simulink model "chap3_7sim"  (Simulink 7.7)
settings: Solver=ode45  SolverMode=SingleTasking  StartTime=0.0  StopTime=10  FixedStep=0.001  RelTol=1e-3
settings Model: Creator=ljk  LastModifiedBy=ljk  ExtModeTrigMode=oneshot  ExtModeArmWhenConnect=off
settings DataIOCC: LimitDataPoints=off
settings OptimizationCC: BlockReduction=off  BooleanDataType=off
settings DebuggingCC: SaveWithParameterizedLinksMsg=none  SignalResolutionControl=TryResolveAllWithWarning  SolverPrmCheckMsg=none  MultiTaskDSMMsg=warning  MultiTaskCondExecSysMsg=none  StrictBusMsg=None
settings HardwareCC: TargetUnknown=on
settings RTWCC: IncludeERTFirstTime=on

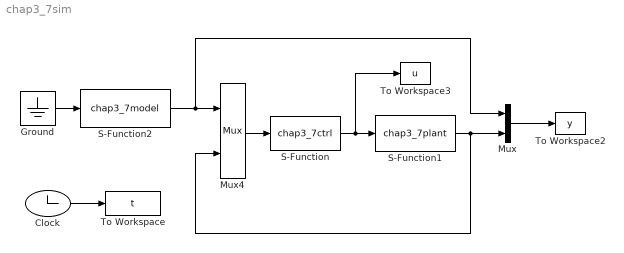
== system chap3_7sim ==
  Clock : Clock
  Ground : Ground
  Mux : Mux  Inputs=2
  Mux4 : Mux  Inputs=2
  S-Function : S-Function  FunctionName=chap3_7ctrl  EnableBusSupport=off
  S-Function1 : S-Function  FunctionName=chap3_7plant  EnableBusSupport=off
  S-Function2 : S-Function  FunctionName=chap3_7model  EnableBusSupport=off
  To Workspace : ToWorkspace  VariableName=t  SampleTime=-1  SaveFormat=Array
  To Workspace2 : ToWorkspace  VariableName=y  SampleTime=-1  SaveFormat=Array
  To Workspace3 : ToWorkspace  VariableName=u  SampleTime=-1  SaveFormat=Array
  wires:
  Mux4/1 -> S-Function/1
  S-Function1/1 -> Mux4/2, Mux/2
  S-Function2/1 -> Mux/1, Mux4/1
  Ground/1 -> S-Function2/1
  Clock/1 -> To Workspace/1
  Mux/1 -> To Workspace2/1
  S-Function/1 -> S-Function1/1, To Workspace3/1
